simulink model "plant"  (R2025b)
settings: Solver=FixedStepAuto  StartTime=0.0  StopTime=inf  RelTol=1e-3  EnableMultiTasking=on
undefined symbols (not defined in the file): LF
libraries: opcualib x13, instrumentseriallib x3, svdutilitieslib x2
settings Model: ExtModeTrigDuration=2  Creator=iarle  LastModifiedBy=iarle
settings OptimizationCC: EnhancedBackFolding=on  PassReuseOutputArgsAs=Individual arguments  ZeroExternalMemoryAtStartup=off  ZeroInternalMemoryAtStartup=off  MaxStackSize=64  OptimizeBlockOrder=speed  DifferentSizesBufferReuse=on  OptimizationCustomize=off  EfficientTunableParamExpr=on
settings DebuggingCC: ParameterTunabilityLossMsg=error
settings HardwareCC: ProdBitPerPointer=32.0  ProdBitPerSizeT=32.0  ProdBitPerPtrDiffT=32.0  ProdLargestAtomicInteger=Long  ProdLargestAtomicFloat=Double  ProdWordSize=32.0  ProdHWDeviceType=ARM Compatible->ARM Cortex
settings SFSimCC: MATLABDynamicMemAlloc=off
settings RTWCC: SystemTargetFile=ert.tlc  HardwareBoard=ESP32-WROOM(Arduino Compatible)  TLCOptions="-aInlineSetEventsForThisBaseRateFcn=TLC_FALSE -aSuppressMultiTaskScheduler=TLC_FALSE  -aRateBasedStepFcn=0"  TemplateMakefile=ert_default_tmf  Toolchain=ESP32  BuildConfiguration=Faster Runs  GPUComputeCapability=3.5  Description=Embedded Coder
settings CodeAppCC: ForceParamTrailComments=on  IgnoreCustomStorageClasses=off  OperatorAnnotations=on  SimulinkDataObjDesc=on  SFDataObjDesc=on  InsertBlockDesc=on
settings ERTTargetCC: ExtModeTransport=3.0  ExtModeStaticAlloc=on  ExtModeAutomaticAllocSize=off  ExtModeStaticAllocSize=65536.0  ExtModeMexFile=ext_xcp  ExtModeIntrfLevel=Level2 - Open  InlinedParameterPlacement=Hierarchical  DynamicArrayContainerType=coder::array  SupportContinuousTime=on  SupportVariableSizeSignals=on

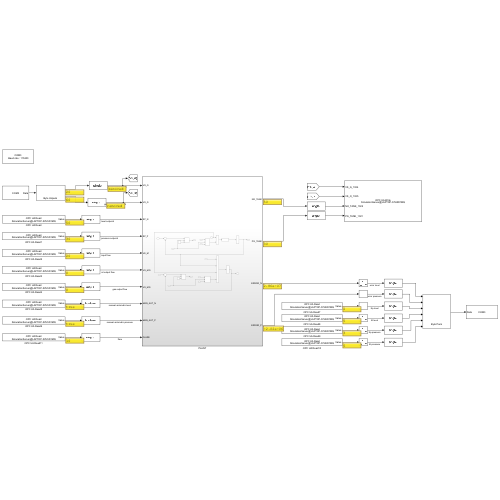
[thumbnail: Simulink's stored preview of the top-level diagram]
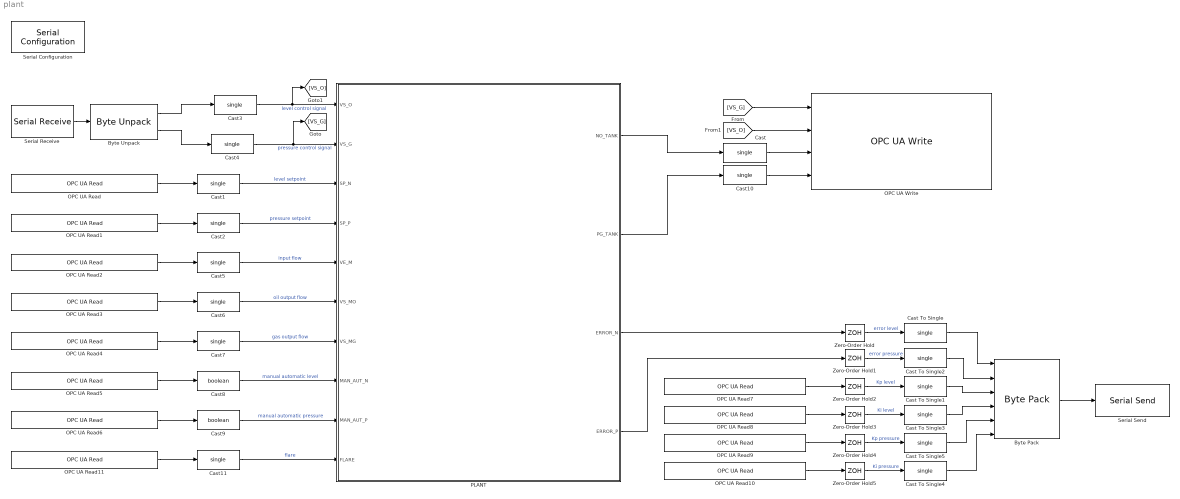
== system plant ==
  Byte Pack : svdutilitieslib/Byte Pack  maskPackedDataType=uint8  datatypes={'single', 'single', 'single', 'single', 'single', 'single'}  byteAlign=4  blockPlatform=arduinoert
  Byte Unpack : svdutilitieslib/Byte Unpack  dimensions={[1], [1]}  datatypes={ 'single', 'single' }  byteAlign=4  blockPlatform=tic2000
      settings: LibrarySourceBlock=c2000lib/Target Communication/Byte Unpack
  Cast{,1..7,10..11} (10 alike) : DataTypeConversion  OutDataTypeStr=single  SaturateOnIntegerOverflow=off  RndMeth=Floor
  Cast To Single{,1..5} (6 alike) : DataTypeConversion  OutDataTypeStr=single  SaturateOnIntegerOverflow=off  RndMeth=Floor
  Cast8 : DataTypeConversion  OutDataTypeStr=boolean  SaturateOnIntegerOverflow=off  RndMeth=Floor
  Cast9 : DataTypeConversion  OutDataTypeStr=boolean  SaturateOnIntegerOverflow=off  RndMeth=Floor
  OPC UA Read : opcualib/OPC UA Read  SelectedServer=SimulationServer@LAPTOP-S7H5D1MQ  ServerList=SimulationServer@LAPTOP-S7H5D1MQ  NodeList={ '1', 'SP_N', '3', '1008', '1' }  ShowQualityPort=off  ShowTimestampPort=off  ShowTimestampPortAs=Seconds since start  SampleTime=-1
  OPC UA Read1 : opcualib/OPC UA Read  SelectedServer=SimulationServer@LAPTOP-S7H5D1MQ  ServerList=SimulationServer@LAPTOP-S7H5D1MQ  NodeList={ '1', 'SP_P', '3', '1014', '1' }  ShowQualityPort=off  ShowTimestampPort=off  ShowTimestampPortAs=Seconds since start  SampleTime=-1
  OPC UA Read10 : opcualib/OPC UA Read  SelectedServer=SimulationServer@LAPTOP-S7H5D1MQ  ServerList=SimulationServer@LAPTOP-S7H5D1MQ  NodeList={ '1', 'I_P', '3', '1016', '1' }  ShowQualityPort=off  ShowTimestampPort=off  ShowTimestampPortAs=Seconds since start  SampleTime=-1
  OPC UA Read11 : opcualib/OPC UA Read  SelectedServer=SimulationServer@LAPTOP-S7H5D1MQ  ServerList=SimulationServer@LAPTOP-S7H5D1MQ  NodeList={ '1', 'FLARE', '3', '1026', '1' }  ShowQualityPort=off  ShowTimestampPort=off  ShowTimestampPortAs=Seconds since start  SampleTime=-1
  OPC UA Read2 : opcualib/OPC UA Read  SelectedServer=SimulationServer@LAPTOP-S7H5D1MQ  ServerList=SimulationServer@LAPTOP-S7H5D1MQ  NodeList={ '1', 'VE_M', '3', '1019', '1' }  ShowQualityPort=off  ShowTimestampPort=off  ShowTimestampPortAs=Seconds since start  SampleTime=-1
  OPC UA Read3 : opcualib/OPC UA Read  SelectedServer=SimulationServer@LAPTOP-S7H5D1MQ  ServerList=SimulationServer@LAPTOP-S7H5D1MQ  NodeList={ '1', 'VS_MO', '3', '1029', '1' }  ShowQualityPort=off  ShowTimestampPort=off  ShowTimestampPortAs=Seconds since start  SampleTime=-1
  OPC UA Read4 : opcualib/OPC UA Read  SelectedServer=SimulationServer@LAPTOP-S7H5D1MQ  ServerList=SimulationServer@LAPTOP-S7H5D1MQ  NodeList={ '1', 'VS_MG', '3', '1028', '1' }  ShowQualityPort=off  ShowTimestampPort=off  ShowTimestampPortAs=Seconds since start  SampleTime=-1
  OPC UA Read5 : opcualib/OPC UA Read  SelectedServer=SimulationServer@LAPTOP-S7H5D1MQ  ServerList=SimulationServer@LAPTOP-S7H5D1MQ  NodeList={ '1', 'MAN_AUT_N', '3', '1012', '1' }  ShowQualityPort=off  ShowTimestampPort=off  ShowTimestampPortAs=Seconds since start  SampleTime=-1
  OPC UA Read6 : opcualib/OPC UA Read  SelectedServer=SimulationServer@LAPTOP-S7H5D1MQ  ServerList=SimulationServer@LAPTOP-S7H5D1MQ  NodeList={ '1', 'MAN_AUT_P', '3', '1017', '1' }  ShowQualityPort=off  ShowTimestampPort=off  ShowTimestampPortAs=Seconds since start  SampleTime=-1
  OPC UA Read7 : opcualib/OPC UA Read  SelectedServer=SimulationServer@LAPTOP-S7H5D1MQ  ServerList=SimulationServer@LAPTOP-S7H5D1MQ  NodeList={ '1', 'P_N', '3', '1011', '1' }  ShowQualityPort=off  ShowTimestampPort=off  ShowTimestampPortAs=Seconds since start  SampleTime=-1
  OPC UA Read8 : opcualib/OPC UA Read  SelectedServer=SimulationServer@LAPTOP-S7H5D1MQ  ServerList=SimulationServer@LAPTOP-S7H5D1MQ  NodeList={ '1', 'I_N', '3', '1013', '1' }  ShowQualityPort=off  ShowTimestampPort=off  ShowTimestampPortAs=Seconds since start  SampleTime=-1
  OPC UA Read9 : opcualib/OPC UA Read  SelectedServer=SimulationServer@LAPTOP-S7H5D1MQ  ServerList=SimulationServer@LAPTOP-S7H5D1MQ  NodeList={ '1', 'P_P', '3', '1015', '1' }  ShowQualityPort=off  ShowTimestampPort=off  ShowTimestampPortAs=Seconds since start  SampleTime=-1
  OPC UA Write : opcualib/OPC UA Write  SelectedServer=SimulationServer@LAPTOP-S7H5D1MQ  ServerList=SimulationServer@LAPTOP-S7H5D1MQ  SampleTime=-1  NodeList={ '1', 'VS_G', '3', '1024', '1'; '2', 'VS_O', '3', '1025', '1'; '3', 'NO_TANK', '3', '1022', '1'; '4', 'PG_TANK', '3', '1021', '1' }
  PLANT : Subsystem
  Serial Configuration : instrumentseriallib/Serial Configuration  Priority=-200000  PortSel=COM3  Port=COM3  ComPort=COM3  BaudRate=115200  DataBits=8  Parity=none  StopBits=1  ByteOrder=little-endian  FlowControl=none  Timeout=10  SimulateUsing=Interpreted execution  BlockInModel=on  aMode=1
      settings: LibrarySourceBlock=c2000lib/Host Communication/Serial Configuration
  Serial Receive : instrumentseriallib/Serial Receive  Priority=1  PortSel=COM3  Port=COM3  ComPort=COM3  DataType=uint8  SaveDataType=uint8  ToggleHeader=on  Header='A'  ToggleDataSize=on  DataSize=[1 8]  ToggleTerminator=on  Terminator=LF ('\n')  CustomTerminator=[]  InputFormat=Row major  EnableBlockingMode=on  ActionDataUnavailable=Output last received value  ActionWhenDataUnavailable=Output last received value  CustomValue=0  SampleTime=0.1  SimulateUsing=Interpreted execution  BlockInModel=on  aMode=1  LibraryInUse=instrumentlib
      settings: LibrarySourceBlock=embeddedtargetslib/Host Communication/Serial Receive
  Serial Send : instrumentseriallib/Serial Send  Priority=1  PortSel=COM3  Port=COM3  ComPort=COM3  Header=['B']  Terminator=LF ('\n')  CustomTerminator=[]  EnableBlockingMode=on  SimulateUsing=Interpreted execution  BlockInModel=on  aMode=1
  Zero-Order Hold{,1..5} (6 alike) : ZeroOrderHold  SampleTime=0.1
  wires:
  Zero-Order Hold/1 -> Cast To Single/1  "error level"
  Byte Pack/1 -> Serial Send/1
  Zero-Order Hold1/1 -> Cast To Single2/1  "error pressure"
  Serial Receive/1 -> Byte Unpack/1
  Byte Unpack/1 -> Cast3/1
  Byte Unpack/2 -> Cast4/1
  PLANT/3(ERROR_N) -> Zero-Order Hold/1
  PLANT/4(ERROR_P) -> Zero-Order Hold1/1
  Cast/1 -> OPC UA Write/3
  OPC UA Read/1 -> Cast1/1
  Cast To Single/1 -> Byte Pack/1
  Cast To Single2/1 -> Byte Pack/2
  Cast To Single1/1 -> Byte Pack/3
  Cast To Single3/1 -> Byte Pack/4
  Cast To Single5/1 -> Byte Pack/5
  Cast To Single4/1 -> Byte Pack/6
  Zero-Order Hold2/1 -> Cast To Single1/1  "Kp level"
  Zero-Order Hold3/1 -> Cast To Single3/1  "Ki level"
  Zero-Order Hold4/1 -> Cast To Single5/1  "Kp pressure"
  Zero-Order Hold5/1 -> Cast To Single4/1  "Ki pressure"
  Cast1/1 -> PLANT/3(SP_N)  "level setpoint"
  OPC UA Read1/1 -> Cast2/1
  Cast2/1 -> PLANT/4(SP_P)  "pressure setpoint"
  Cast3/1 -> [VS_O], PLANT/1(VS_O)  "level control signal"
  Cast4/1 -> [VS_G], PLANT/2(VS_G)  "pressure control signal"
  Cast5/1 -> PLANT/5(VE_M)  "input flow"
  OPC UA Read2/1 -> Cast5/1
  OPC UA Read3/1 -> Cast6/1
  Cast6/1 -> PLANT/6(VS_MO)  "oil output flow"
  OPC UA Read4/1 -> Cast7/1
  Cast7/1 -> PLANT/7(VS_MG)  "gas output flow"
  Cast8/1 -> PLANT/8(MAN_AUT_N)  "manual automatic level"
  OPC UA Read5/1 -> Cast8/1
  OPC UA Read6/1 -> Cast9/1
  Cast9/1 -> PLANT/9(MAN_AUT_P)  "manual automatic pressure"
  OPC UA Read7/1 -> Zero-Order Hold2/1
  OPC UA Read8/1 -> Zero-Order Hold3/1
  OPC UA Read9/1 -> Zero-Order Hold4/1
  OPC UA Read10/1 -> Zero-Order Hold5/1
  PLANT/1(NO_TANK) -> Cast/1
  PLANT/2(PG_TANK) -> Cast10/1
  Cast11/1 -> PLANT/10(FLARE)  "flare"
  OPC UA Read11/1 -> Cast11/1
  Cast10/1 -> OPC UA Write/4
  [VS_G] -> OPC UA Write/1
  [VS_O] -> OPC UA Write/2

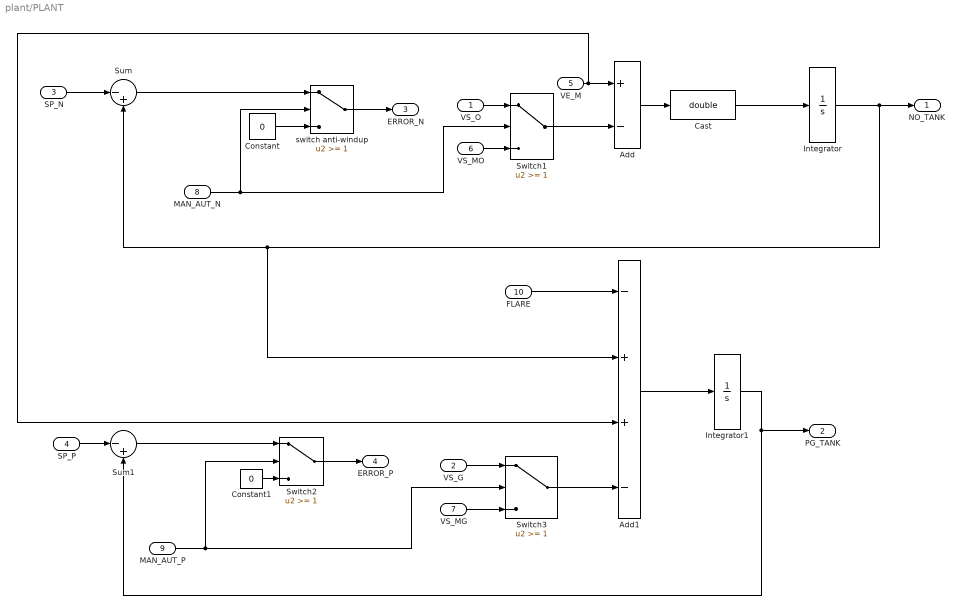
== system plant/PLANT ==
  VS_O : Inport
  VS_G : Inport  Port=2
  SP_N : Inport  Port=3
  SP_P : Inport  Port=4
  VE_M : Inport  Port=5
  VS_MO : Inport  Port=6
  VS_MG : Inport  Port=7
  MAN_AUT_N : Inport  Port=8
  MAN_AUT_P : Inport  Port=9
  FLARE : Inport  Port=10
  Add : Sum  Inputs=+-
  Add1 : Sum  Inputs=-++-
  Cast : DataTypeConversion  OutDataTypeStr=double  SaturateOnIntegerOverflow=off  RndMeth=Floor
  Constant : Constant  Value=0
  Constant1 : Constant  Value=0
  Integrator : Integrator  LimitOutput=on  UpperSaturationLimit=100  LowerSaturationLimit=0
  Integrator1 : Integrator  LimitOutput=on  UpperSaturationLimit=100  LowerSaturationLimit=0
  Sum : Sum  Inputs=|-+
  Sum1 : Sum  Inputs=|-+
  Switch1 : Switch  Threshold=1  SaturateOnIntegerOverflow=off  InputSameDT=off
  Switch2 : Switch  Threshold=1  SaturateOnIntegerOverflow=off  InputSameDT=off
  Switch3 : Switch  Threshold=1  SaturateOnIntegerOverflow=off  InputSameDT=off
  switch anti-windup : Switch  Threshold=1  SaturateOnIntegerOverflow=off  InputSameDT=off
  NO_TANK : Outport
  PG_TANK : Outport  Port=2
  ERROR_N : Outport  Port=3
  ERROR_P : Outport  Port=4
  wires:
  SP_P/1 -> Sum1/1
  Constant1/1 -> Switch2/3
  MAN_AUT_P/1 -> Switch2/2, Switch3/2
  Sum1/1 -> Switch2/1
  Integrator/1 -> NO_TANK/1, Add1/2, Sum/2
  Switch3/1 -> Add1/4
  VS_MG/1 -> Switch3/3
  Sum/1 -> switch anti-windup/1
  Constant/1 -> switch anti-windup/3
  Add1/1 -> Integrator1/1
  MAN_AUT_N/1 -> Switch1/2, switch anti-windup/2
  VS_MO/1 -> Switch1/3
  Switch2/1 -> ERROR_P/1
  VS_G/1 -> Switch3/1
  Switch1/1 -> Add/2
  VE_M/1 -> Add/1, Add1/3
  SP_N/1 -> Sum/1
  Integrator1/1 -> PG_TANK/1, Sum1/2
  switch anti-windup/1 -> ERROR_N/1
  VS_O/1 -> Switch1/1
  FLARE/1 -> Add1/1
  Add/1 -> Cast/1
  Cast/1 -> Integrator/1
